simulink model "State_Machine_Harness2"  (R2022b)
settings: Solver=FixedStepDiscrete  StartTime=0.0  StopTime=10  RelTol=1e-3
undefined symbols (not defined in the file): BMS_State_Enum
settings Model: DataDictionary=DD_State_Machine.sldd  Creator=cpatel  LastModifiedBy=cpatel
settings SolverCC: AlgebraicLoopSolver=TrustRegion  PositivePriorityOrder=on  AutoInsertRateTranBlk=on
settings DataIOCC: ExternalInput=Battery  SaveOutput=off  SaveTime=off  SignalLoggingName=logsOut
settings OptimizationCC: BlockReduction=off  DefaultParameterBehavior=Inlined  UseFloatMulNetSlope=on  DefaultUnderspecifiedDataType=single  EnhancedBackFolding=on  PassReuseOutputArgsAs=Individual arguments  ZeroExternalMemoryAtStartup=off  ZeroInternalMemoryAtStartup=off  EfficientFloat2IntCast=on  MaxStackSize=64  OptimizeBlockOrder=speed  DifferentSizesBufferReuse=on  OptimizationCustomize=off  EfficientTunableParamExpr=on
settings DebuggingCC: SignalInfNanChecking=error  SaveWithParameterizedLinksMsg=none  CheckExecutionContextPreStartOutputMsg=on  IntegerOverflowMsg=error  ParameterPrecisionLossMsg=none  ParameterTunabilityLossMsg=error  UnconnectedInputMsg=warning  UnconnectedOutputMsg=warning  UnconnectedLineMsg=warning  AssertControl=DisableAll  PregeneratedLibrarySubsystemCodeDiagnostic=none  SFUnexpectedBacktrackingDiag=warning  SFNoUnconditionalDefaultTransitionDiag=warning  SFExecutionAtInitializationDiag=none  SFMachineParentedDataDiag=warning  ArithmeticOperatorsInVariantConditions=warning
settings HardwareCC: ProdBitPerPointer=32  ProdBitPerSizeT=32  ProdBitPerPtrDiffT=32  ProdLargestAtomicInteger=Long  ProdLargestAtomicFloat=Double  ProdWordSize=32  ProdHWDeviceType=ARM Compatible->ARM Cortex-M
settings ModelReferenceCC: EnableRefExpFcnMdlSchedulingChecks=on  ModelReferenceNumInstancesAllowed=Single  PropagateSignalLabelsOutOfModel=off
settings SFSimCC: SimUseLocalCustomCode=off  MATLABDynamicMemAlloc=off  CustomCodeUndefinedFunction=UseInterfaceOnly
settings RTWCC: Description=Embedded Coder  SystemTargetFile=ert.tlc  GenCodeOnly=on  TemplateMakefile=ert_default_tmf  GenerateReport=on  RTWUseLocalCustomCode=off  BuildConfiguration=Faster Runs  CodeExecutionProfiling=on  DLArmComputeVersion=19.05
settings CodeAppCC: ForceParamTrailComments=on  IgnoreCustomStorageClasses=off  MaxIdLength=51  OperatorAnnotations=on  SimulinkDataObjDesc=on  SFDataObjDesc=on  MangleLength=4  InsertBlockDesc=on  ReqsInCode=on
settings ERTTargetCC: TargetLangStandard=C99 (ISO)  CodeReplacementLibrary=GNU C99 extensions  UtilityFuncGeneration=Shared location  GenerateFullHeader=off  ERTCustomFileBanners=off  SupportAbsoluteTime=off  SupportNonFinite=off  SupportComplex=off  SupportVariableSizeSignals=on  InlinedParameterPlacement=NonHierarchical  RootIOFormat=Structure reference  ERTCustomFileTemplate=example_file_process.tlc
settings ConfigComp: CovEnable=on  CovScope=ReferencedModels  CovIncludeTopModel=off  CovSaveName=sltest_covdata  CovMetricSettings=dcmwe  CovEnableCumulative=off  CovSaveCumulativeToWorkspaceVar=on  CovSaveSingleToWorkspaceVar=on  CovSaveOutputData=off  CovOutputDir=C:\Users\cpatel\Documents\BatteryManagementSystem\slcov_output\State_Machine  CovDataFileName=State_Machine_cvdata_8.cvt  CovModelRefEnable=on  DVMode=DesignErrorDetection  DVMaxProcessTime=7000  DVTestSuiteOptimization=Auto  DVDetectDeadLogic=on  DVDetectIntegerOverflow=off  DVRebuildModelRepresentation=Always

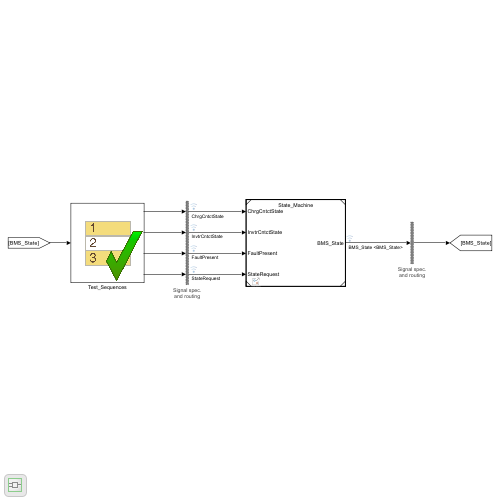
[thumbnail: Simulink's stored preview of the top-level diagram]
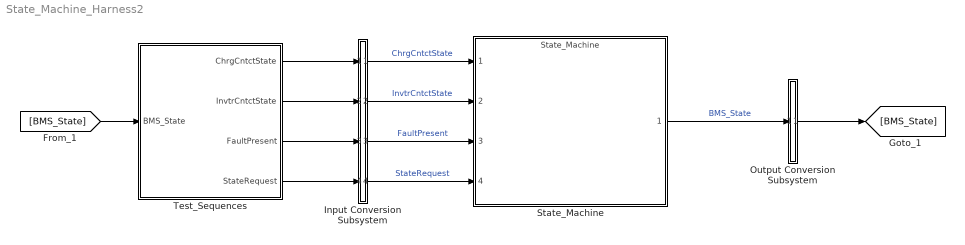
== system State_Machine_Harness2 ==
  Input Conversion Subsystem : Subsystem  Tag=__SLT_ICS__  Description=|
      | Signal spec.
      | and routing
      settings: AttributesFormatString=%<Description>
  Output Conversion Subsystem : Subsystem  Tag=__SLT_OCS__  Description=|
      | Signal spec.
      | and routing
      settings: AttributesFormatString=%<Description>
  State_Machine : ModelReference  ModelNameDialog=State_Machine  SimulationMode=Normal  ModelReferenceVersion=5.1
  Test_Sequences : Test Sequence  TreatAsAtomicUnit=on
  wires:
  Test_Sequences/1(ChrgCntctState) -> Input Conversion Subsystem/1(Inport_1)
  Test_Sequences/2(InvtrCntctState) -> Input Conversion Subsystem/2(Inport_2)
  Test_Sequences/3(FaultPresent) -> Input Conversion Subsystem/3(Inport_3)
  Test_Sequences/4(StateRequest) -> Input Conversion Subsystem/4(Inport_4)
  [BMS_State] -> Test_Sequences/1(BMS_State)
  Output Conversion Subsystem/1(Outport_1) -> [BMS_State]
  Input Conversion Subsystem/1(Outport_1) -> State_Machine/1  "ChrgCntctState"
  Input Conversion Subsystem/2(Outport_2) -> State_Machine/2  "InvtrCntctState"
  Input Conversion Subsystem/3(Outport_3) -> State_Machine/3  "FaultPresent"
  Input Conversion Subsystem/4(Outport_4) -> State_Machine/4  "StateRequest"
  State_Machine/1 -> Output Conversion Subsystem/1(Inport_1)  "BMS_State"

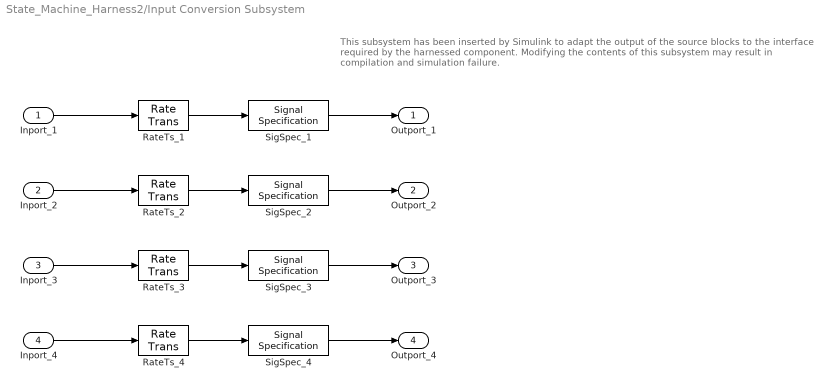
== system State_Machine_Harness2/Input Conversion Subsystem ==
  note: This subsystem has been inserted by Simulink to adapt the output of the source blocks to the interface required by the harnessed component.
      |  Modifying the contents of this subsystem may result in compilation and simulation failure.
  Inport_1 : Inport
  Inport_2 : Inport  Port=2
  Inport_3 : Inport  Port=3
  Inport_4 : Inport  Port=4
  RateTs_{1..4} (4 alike) : RateTransition  OutPortSampleTime=0.1
  SigSpec_1 : SignalSpecification  OutDataTypeStr=Enum: Contact  Dimensions=[1]  SampleTime=0.1
  SigSpec_2 : SignalSpecification  OutDataTypeStr=Enum: Contact  Dimensions=[1]  SampleTime=0.1
  SigSpec_3 : SignalSpecification  OutDataTypeStr=boolean  Dimensions=[1]  SampleTime=0.1
  SigSpec_4 : SignalSpecification  OutDataTypeStr=Enum: SRE  Dimensions=[1]  SampleTime=0.1
  Outport_1 : Outport
  Outport_2 : Outport  Port=2
  Outport_3 : Outport  Port=3
  Outport_4 : Outport  Port=4
  wires:
  SigSpec_1/1 -> Outport_1/1
  RateTs_1/1 -> SigSpec_1/1
  Inport_1/1 -> RateTs_1/1
  SigSpec_2/1 -> Outport_2/1
  RateTs_2/1 -> SigSpec_2/1
  Inport_2/1 -> RateTs_2/1
  SigSpec_3/1 -> Outport_3/1
  RateTs_3/1 -> SigSpec_3/1
  Inport_3/1 -> RateTs_3/1
  SigSpec_4/1 -> Outport_4/1
  RateTs_4/1 -> SigSpec_4/1
  Inport_4/1 -> RateTs_4/1

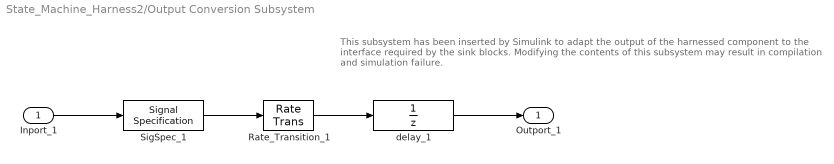
== system State_Machine_Harness2/Output Conversion Subsystem ==
  note: This subsystem has been inserted by Simulink to adapt the output of the harnessed component to the interface required by the sink blocks.
      |  Modifying the contents of this subsystem may result in compilation and simulation failure.
  Inport_1 : Inport
  Rate_Transition_1 : RateTransition  InitialCondition=BMS_State_Enum.BMS_Standby  OutPortSampleTimeOpt=Inherit
  SigSpec_1 : SignalSpecification  OutDataTypeStr=Enum: BMS_State_Enum  Dimensions=[1]  SampleTime=0.1
  delay_1 : UnitDelay  InitialCondition=BMS_State_Enum.BMS_Standby  SampleTime=-1
  Outport_1 : Outport
  wires:
  Inport_1/1 -> SigSpec_1/1
  SigSpec_1/1 -> Rate_Transition_1/1
  Rate_Transition_1/1 -> delay_1/1
  delay_1/1 -> Outport_1/1

== stateflow chart State_Machine_Harness2/Test_Sequences ==
  state Standby
    state Init
      %% Initialize data outputs.
      ChrgCntctState = Contact.Init;
      InvtrCntctState = Contact.Init;
      FaultPresent = false;
      StateRequest = SRE.Standby;
      verify(BMS_State == BMS_State_Enum.BMS_Standby, 'Initialize to BMS State.');
    (default) -> Standby.Init
  state StandbyToFault
    state Init
      %% Initialize data outputs.
      ChrgCntctState = Contact.Init;
      InvtrCntctState = Contact.Init;
      FaultPresent = false;
      StateRequest = SRE.Standby;
    state Insert_Fault
      FaultPresent = true;
    state CheckForFaultState
      verify(BMS_State == BMS_State_Enum.BMS_Fault,'Verify Standby to Fault Transition');
    (default) -> StandbyToFault.Init
    StandbyToFault.Init -> Insert_Fault : [
        | after(5,sec)
        | ]
    Insert_Fault -> StandbyToFault.CheckForFaultState : [
        | after(100,msec)
        | ]
  state Charging
    state Init
      %% Initialize data outputs.
      ChrgCntctState = Contact.Init;
      InvtrCntctState = Contact.Init;
      FaultPresent = false;
      StateRequest = SRE.Charging;
      verify(BMS_State ~= BMS_State_Enum.BMS_Charging, 'BMS shall not transition to Charging State when charger contactors are NOT Close');
    state CloseChargerContactors
      ChrgCntctState = Contact.Close;
    state CheckForChargingState
      verify(BMS_State == BMS_State_Enum.BMS_Charging,'BMS shall transition to Charging State when charger contactors are Close');
    state OpenChargerContactors
      ChrgCntctState = Contact.Open;
    state CheckForStandbyState
      verify(BMS_State == BMS_State_Enum.BMS_Standby,'BMS shall transition to Standby State when charger contactors are Open');
    (default) -> Charging.Init
    Charging.Init -> Charging.CloseChargerContactors : [
        | after(2,sec)
        | ]
    Charging.CloseChargerContactors -> Charging.CheckForChargingState : [
        | after(100,msec)
        | ]
    Charging.CheckForChargingState -> OpenChargerContactors : [
        | after(2, sec)
        | ]
    OpenChargerContactors -> Charging.CheckForStandbyState : [
        | after(100,msec)
        | ]
  state ChargingToFault
    state Init
      %% Initialize data outputs.
      ChrgCntctState = Contact.Init;
      InvtrCntctState = Contact.Init;
      FaultPresent = false;
      StateRequest = SRE.Charging;
      verify(BMS_State ~= BMS_State_Enum.BMS_Charging, 'BMS shall not transition to Charging State when charger contactors are NOT Close');
    state CloseChargerContactors
      ChrgCntctState = Contact.Close;
    state CheckForChargingState
      verify(BMS_State == BMS_State_Enum.BMS_Charging,'BMS shall transition to Charging State when charger contactors are Close');
    state InsertFault
      FaultPresent = true;
    state CheckForFaultState
      verify(BMS_State == BMS_State_Enum.BMS_Fault,'BMS shall transition to Fault State when any fault is present');
    (default) -> ChargingToFault.Init
    ChargingToFault.Init -> ChargingToFault.CloseChargerContactors : [
        | after(2,sec)
        | ]
    ChargingToFault.CloseChargerContactors -> ChargingToFault.CheckForChargingState : [
        | after(100,msec)
        | ]
    ChargingToFault.CheckForChargingState -> ChargingToFault.InsertFault : [
        | after(2, sec)
        | ]
    ChargingToFault.InsertFault -> ChargingToFault.CheckForFaultState : [
        | after(100,msec)
        | ]
  state Driving
    state Init
      %% Initialize data outputs.
      ChrgCntctState = Contact.Init;
      InvtrCntctState = Contact.Init;
      FaultPresent = false;
      StateRequest = SRE.Driving;
      verify(BMS_State ~= BMS_State_Enum.BMS_Driving, 'BMS shall not transition to Driving State when Invertor contactors are NOT Close');
    state CloseInvertorContactors
      InvtrCntctState = Contact.Close;
    state CheckForDrivingState
      verify(BMS_State == BMS_State_Enum.BMS_Driving,'BMS shall transition to Driving State when Invertor contactors are Close');
    state OpenInvertorContactors
      InvtrCntctState = Contact.Open;
    state CheckForStandbyState
      verify(BMS_State == BMS_State_Enum.BMS_Standby,'BMS shall transition to Standby State when Invertor contactors are Open');
    (default) -> Driving.Init
    Driving.Init -> Driving.CloseInvertorContactors : [
        | after(2,sec)
        | ]
    Driving.CloseInvertorContactors -> Driving.CheckForDrivingState : [
        | after(100,msec)
        | ]
    Driving.CheckForDrivingState -> OpenInvertorContactors : [
        | after(2, sec)
        | ]
    OpenInvertorContactors -> Driving.CheckForStandbyState : [
        | after(100,msec)
        | ]
  state DrivingToFault
    state Init
      %% Initialize data outputs.
      ChrgCntctState = Contact.Init;
      InvtrCntctState = Contact.Init;
      FaultPresent = false;
      StateRequest = SRE.Driving;
      verify(BMS_State ~= BMS_State_Enum.BMS_Driving, 'BMS shall not transition to Driving State when Invertor contactors are NOT Close');
    state CloseInvertorContactors
      InvtrCntctState = Contact.Close;
    state CheckForDrivingState
      verify(BMS_State == BMS_State_Enum.BMS_Driving,'BMS shall transition to Driving State when Invertor contactors are Close');
    state InsertFault
      FaultPresent= true;
    state CheckForFaultState
      verify(BMS_State == BMS_State_Enum.BMS_Fault,'BMS shall transition to Fault State when any fault is present');
    (default) -> DrivingToFault.Init
    DrivingToFault.Init -> DrivingToFault.CloseInvertorContactors : [
        | after(2,sec)
        | ]
    DrivingToFault.CloseInvertorContactors -> DrivingToFault.CheckForDrivingState : [
        | after(100,msec)
        | ]
    DrivingToFault.CheckForDrivingState -> DrivingToFault.InsertFault : [
        | after(2, sec)
        | ]
    DrivingToFault.InsertFault -> DrivingToFault.CheckForFaultState : [
        | after(100,msec)
        | ]
  state ChargingToStandby
    state Init
      %% Initialize data outputs.
      ChrgCntctState = Contact.Init;
      InvtrCntctState = Contact.Init;
      FaultPresent = false;
      StateRequest = SRE.Charging;
      verify(BMS_State ~= BMS_State_Enum.BMS_Charging, 'BMS shall not transition to Charging State when charger contactors are NOT Close');
    state CloseChargerContactors
      ChrgCntctState = Contact.Close;
    state CheckForChargingState
      verify(BMS_State == BMS_State_Enum.BMS_Charging,'BMS shall transition to Charging State when charger contactors are Close');
    state StandbyRequest
      StateRequest = SRE.Standby;
    state CheckForStandbyState
      verify(BMS_State == BMS_State_Enum.BMS_Standby,'BMS shall transition to Stanby State when StateRequest is Standby');
    (default) -> ChargingToStandby.Init
    ChargingToStandby.Init -> ChargingToStandby.CloseChargerContactors : [
        | after(2,sec)
        | ]
    ChargingToStandby.CloseChargerContactors -> ChargingToStandby.CheckForChargingState : [
        | after(100,msec)
        | ]
    ChargingToStandby.CheckForChargingState -> ChargingToStandby.StandbyRequest : [
        | after(2, sec)
        | ]
    ChargingToStandby.StandbyRequest -> ChargingToStandby.CheckForStandbyState : [
        | after(100,msec)
        | ]
  state DrivingtoStandby
    state Init
      %% Initialize data outputs.
      ChrgCntctState = Contact.Init;
      InvtrCntctState = Contact.Init;
      FaultPresent = false;
      StateRequest = SRE.Driving;
      verify(BMS_State ~= BMS_State_Enum.BMS_Driving, 'BMS shall not transition to Driving State when Invertor contactors are NOT Close');
    state CloseInvertorContactors
      InvtrCntctState = Contact.Close;
    state CheckForDrivingState
      verify(BMS_State == BMS_State_Enum.BMS_Driving,'BMS shall transition to Driving State when Invertor contactors are Close');
    state StandbyRequest
      StateRequest = SRE.Standby;
    state CheckForStandbyState
      verify(BMS_State == BMS_State_Enum.BMS_Standby,'BMS shall transition to Stanby State when StateRequest is Standby');
    (default) -> DrivingtoStandby.Init
    DrivingtoStandby.Init -> DrivingtoStandby.CloseInvertorContactors : [
        | after(2,sec)
        | ]
    DrivingtoStandby.CloseInvertorContactors -> DrivingtoStandby.CheckForDrivingState : [
        | after(100,msec)
        | ]
    DrivingtoStandby.CheckForDrivingState -> DrivingtoStandby.StandbyRequest : [
        | after(2, sec)
        | ]
    DrivingtoStandby.StandbyRequest -> DrivingtoStandby.CheckForStandbyState : [
        | after(100,msec)
        | ]
  (default) -> Standby [order 1] : [Active_Scenario_Index == 1]
  (default) -> StandbyToFault [order 2] : [Active_Scenario_Index == 2]
  (default) -> Charging [order 3] : [Active_Scenario_Index == 3]
  (default) -> ChargingToFault [order 4] : [Active_Scenario_Index == 4]
  (default) -> Driving [order 5] : [Active_Scenario_Index == 5]
  (default) -> DrivingToFault [order 6] : [Active_Scenario_Index == 6]
  (default) -> ChargingToStandby [order 7] : [Active_Scenario_Index == 7]
  (default) -> DrivingtoStandby [order 8] : {assert(Active_Scenario_Index == 8,'The value of Scenario Parameter ''Active_Scenario_Index'' is not valid. Use the index of the scenario to specify it.')}
  data: BMS_State input Enum: BMS_State_Enum size=[1]; ChrgCntctState output Enum: Contact size=[1]; InvtrCntctState output Enum: Contact size=[1]; FaultPresent output boolean size=[1]; StateRequest output Enum: SRE size=[1]; Active_Scenario_Index parameter =8
